simulink model "simulation_model_constcurrent"  (R2024b)
settings: Solver=VariableStepAuto  StartTime=0.0  StopTime=100  MaxStep=1/60  RelTol=1e-3  EnableMultiTasking=on
values from neighbouring files (symbols this model uses):
  c_f = c_f*Cb    [fun00_GFL_pu_2_normial.m]    (also in fun00_GFM_pu_2_normial.m)
  fb = 60    [case_data.m]    (also in sim_m_case1.m; sim_m_case1_bench.m; sim_m_case2.m; sim_m_case2_bench.m)
  ki_i = ki_i_pu*Vb_p_ph/Ib_p_ph    [fun00_GFL_pu_2_normial.m]    (also in fun00_GFM_pu_2_normial.m)
  ki_p = ki_p_pu/Sb*Ib_p_ph    [fun00_GFL_pu_2_normial.m]
  ki_pll = ki_pll/Vb_p_ph    [fun00_GFL_pu_2_normial.m]
  ki_q = ki_q_pu/Sb*Ib_p_ph    [fun00_GFL_pu_2_normial.m]
  kp_i = kp_i_pu*Vb_p_ph/Ib_p_ph    [fun00_GFL_pu_2_normial.m]    (also in fun00_GFM_pu_2_normial.m)
  kp_p = kp_p_pu/Sb*Ib_p_ph    [fun00_GFL_pu_2_normial.m]
  kp_pll = kp_pll/Vb_p_ph    [fun00_GFL_pu_2_normial.m]
  kp_q = kp_q_pu/Sb*Ib_p_ph    [fun00_GFL_pu_2_normial.m]
  l_f = l_f*Lb    [fun00_GFL_pu_2_normial.m]    (also in fun00_GFM_pu_2_normial.m)
  line = mpc.line    [sim_m_case1.m]    (also in sim_m_case1_bench.m; sim_m_case2.m = mpc.line*1.1; sim_m_case2_bench.m = mpc.line*1.1; sim_m_case2_sparse.m = mpc.line*1.1)
  pset = p_set_pu*Sb    [fun00_GFL_pu_2_normial.m]
  qset = q_set_pu*Sb    [fun00_GFL_pu_2_normial.m]
  r_f = r_f*Zb    [fun00_GFL_pu_2_normial.m]    (also in fun00_GFM_pu_2_normial.m)
  Sb = 100*10^6    (= 100000000)    [sim_m_case1.m]    (also in sim_m_case1_bench.m; sim_m_case2.m; sim_m_case2_bench.m; sim_m_case2_sparse.m)
  t_gfl = 35    [sim_m_case1.m]    (also in sim_m_case1_bench.m = 30; sim_m_case2.m; sim_m_case2_bench.m = 30; sim_m_case2_sparse.m)
  t_gfm = 30    [sim_m_case1.m]    (also in sim_m_case1_bench.m; sim_m_case2.m; sim_m_case2_bench.m; sim_m_case2_sparse.m)
  trans_l = mpc.trans_l    [sim_m_case1.m]    (also in sim_m_case1_bench.m; sim_m_case2.m; sim_m_case2_bench.m; sim_m_case2_sparse.m)
  Vb_gfm = 20*10^3    (= 20000)    [sim_m_case1.m]    (also in sim_m_case1_bench.m; sim_m_case2.m; sim_m_case2_bench.m; sim_m_case2_sparse.m)
  Vb_h = 230*10^3    (= 230000)    [sim_m_case1.m]    (also in sim_m_case1_bench.m; sim_m_case2.m; sim_m_case2_bench.m; sim_m_case2_sparse.m)
  Vdc = 3*Vb_p_ph    [fun00_GFL_pu_2_normial.m]    (also in fun00_GFM_pu_2_normial.m)
  wb = 2*pi*fb    (= 376.991118431)    [case_data.m]    (also in sim_m_case1.m; sim_m_case1_bench.m; sim_m_case2.m; sim_m_case2_bench.m)
undefined symbols (not defined in the file or in its folder): c_f_gfm, d_gfl, D_p_gfm, D_p_gfm_s, D_q_gfm, DiscIntNeverNeededParam, Init, Init_GFL, J_gfm, ki_i_gfm, ki_pll_s, ki_vc_gfm, kp_i_gfm, kp_pll_s, kp_vc_gfm, l_f_gfm, P_set_gfm, Q_set_gfm, r_f_gfm, Vb, Vdc_gfm, VSM
libraries: spsThreePhaseVIMeasurementLib x52, spsabctodq0Lib x48, slpidlib x42, spsThreePhaseSeriesRLCBranchLib x36, spsFirstOrderFilterLib x16, spsThreePhaseTransformerTwoWindingsLib x9, spsGroundLib x9, spsPowerPositiveSequenceLib x9, spsdq0toabcLib x9, spsUniversalBridgeLib x9, spsDCVoltageSourceLib x9, spsThreePhaseSourceLib x5
(part 7 of 8)

== system simulation_model_constcurrent/Area 3/INVERTER 7/GFM7/Current Lopp ==
  Vodq : Inport
  Icdq : Inport  Port=2
  i_ref_dq : Inport  Port=3
  theta : Inport  Port=4
  Demux : Demux  Outputs=2
  Demux1 : Demux  Outputs=2
  Demux4 : Demux  Outputs=2
  Gain : Gain  Gain=2/Vdcnorm
  Mux1 : Mux  Inputs=3
  Mux3 : Mux  Inputs=2
  Mux4 : Mux  Inputs=2
  PID Controller2 : slpidlib/PID Controller  Controller=PI  Form=Parallel  TimeDomain=Continuous-time  UseExternalTs=off  SampleTime=-1  IntegratorMethod=Forward Euler  FilterMethod=Forward Euler  ControllerParametersSource=internal  P=Current_P  I=Current_I  UseKiTs=off  D=0  UseExternalDerivativeSource=off  N=100  UseFilter=on  TunerSelectOption=Transfer Function Based (PID Tuner App)  InitialConditionSource=internal  InitialConditionForIntegrator=InitialV.Vcd-InitialV.Vod  InitialConditionForFilter=0  DifferentiatorICPrevScaledInput=0  ExternalReset=none  TrackingMode=off  Kt=1  LimitOutput=off  SatLimitsSource=internal  UpperSaturationLimit=inf  LowerSaturationLimit=-inf  LinearizeAsGain=on  AntiWindupMode=none  Kb=1  LimitIntegrator=off  UpperIntegratorSaturationLimit=inf  LowerIntegratorSaturationLimit=-inf  POutMin=[]  POutMax=[]  IOutMin=[]  IOutMax=[]  DOutMin=[]  DOutMax=[]  NOutMin=[]  NOutMax=[]  SumOutMin=[]  SumOutMax=[]  SaturationOutMin=[]  SaturationOutMax=[]  PParamMin=[]  PParamMax=[]  IParamMin=[]  IParamMax=[]  DParamMin=[]  DParamMax=[]  NParamMin=[]  NParamMax=[]  KbParamMin=[]  KbParamMax=[]  KtParamMin=[]  KtParamMax=[]  KbOutMin=[]  KbOutMax=[]  KtOutMin=[]  KtOutMax=[]  IntegratorOutMin=[]  IntegratorOutMax=[]  FilterOutMin=[]  FilterOutMax=[]  SumI1OutMin=[]  SumI1OutMax=[]  SumI2OutMin=[]  SumI2OutMax=[]  SumI3OutMin=[]  SumI3OutMax=[]  SumI4OutMin=[]  SumI4OutMax=[]  SumDOutMin=[]  SumDOutMax=[]  DifferentiatorOutMin=[]  DifferentiatorOutMax=[]  FilterDiffOutCoefMin=[]  FilterDiffOutCoefMax=[]  ReciprocalOutMin=[]  ReciprocalOutMax=[]  SumDenOutMin=[]  SumDenOutMax=[]  SumNumOutMin=[]  SumNumOutMax=[]  DivideOutMin=[]  DivideOutMax=[]  UdiffTsProdOutMin=[]  UdiffTsProdOutMax=[]  NTsProdOutMin=[]  NTsProdOutMax=[]  UintegralTsProdOutMin=[]  UintegralTsProdOutMax=[]  UngainTsProdOutMin=[]  UngainTsProdOutMax=[]  ClampingZeroOutDataTypeStr=Inherit: Inherit via back propagation  ClampingZeroOutMin=[]  ClampingZeroOutMax=[]  FilterDenConstantOutDataTypeStr=Inherit: Inherit via back propagation  FilterDenConstantOutMin=[]  FilterDenConstantOutMax=[]  PCopyOutDataTypeStr=Inherit: Inherit via back propagation  PCopyOutMin=[]  PCopyOutMax=[]  NCopyOutDataTypeStr=Inherit: Inherit via back propagation  NCopyOutMin=[]  NCopyOutMax=[]  IntegratorContinuousStateAttributes=''  IntegratorStateMustResolveToSignalObject=off  IntegratorRTWStateStorageClass=Auto  FilterContinuousStateAttributes=''  FilterStateMustResolveToSignalObject=off  FilterRTWStateStorageClass=Auto  ParallelPVariant=InternalParameters  IdealPVariant=Disabled  IVariant=InternalParameters  DVariant=Disabled  IntegratorVariant=Continuous  SatVariant=Disabled  AWVariant=Passthrough  PCopyVariant=Disabled  TRVariant=Disabled  FdbkBlocksVariant=Forward  IdealPFdbkVariant=Disabled  SatFdbkVariant=Disabled  DerivativeFilterVariant=Disabled  NVariant=Disabled  NCopyVariant=Disabled_SignalSpec  FilterICVariant=Disabled  IntegratorICVariant=InternalICs  ExternalResetVariant=Disabled  TRSumVariant=Passthrough  SumFdbkVariant=Disabled  SumVariant=Sum_PI  TsampFilterVariant=InternalTs  TsampNgainVariant=Passthrough  TsampIntegralVariant=Disabled_SignalSpec  ExternalSaturationOutDataTypeStr=Inherit: Same as second input  DerivativeSourceVariant=Disabled  PreIntVariant=InternalPreInt
  PID Controller3 : slpidlib/PID Controller  Controller=PI  Form=Parallel  TimeDomain=Continuous-time  UseExternalTs=off  SampleTime=-1  IntegratorMethod=Forward Euler  FilterMethod=Forward Euler  ControllerParametersSource=internal  P=Current_P  I=Current_I  UseKiTs=off  D=0  UseExternalDerivativeSource=off  N=100  UseFilter=on  TunerSelectOption=Transfer Function Based (PID Tuner App)  InitialConditionSource=internal  InitialConditionForIntegrator=InitialV.Vcq-InitialV.Voq  InitialConditionForFilter=0  DifferentiatorICPrevScaledInput=0  ExternalReset=none  TrackingMode=off  Kt=1  LimitOutput=off  SatLimitsSource=internal  UpperSaturationLimit=inf  LowerSaturationLimit=-inf  LinearizeAsGain=on  AntiWindupMode=none  Kb=1  LimitIntegrator=off  UpperIntegratorSaturationLimit=inf  LowerIntegratorSaturationLimit=-inf  POutMin=[]  POutMax=[]  IOutMin=[]  IOutMax=[]  DOutMin=[]  DOutMax=[]  NOutMin=[]  NOutMax=[]  SumOutMin=[]  SumOutMax=[]  SaturationOutMin=[]  SaturationOutMax=[]  PParamMin=[]  PParamMax=[]  IParamMin=[]  IParamMax=[]  DParamMin=[]  DParamMax=[]  NParamMin=[]  NParamMax=[]  KbParamMin=[]  KbParamMax=[]  KtParamMin=[]  KtParamMax=[]  KbOutMin=[]  KbOutMax=[]  KtOutMin=[]  KtOutMax=[]  IntegratorOutMin=[]  IntegratorOutMax=[]  FilterOutMin=[]  FilterOutMax=[]  SumI1OutMin=[]  SumI1OutMax=[]  SumI2OutMin=[]  SumI2OutMax=[]  SumI3OutMin=[]  SumI3OutMax=[]  SumI4OutMin=[]  SumI4OutMax=[]  SumDOutMin=[]  SumDOutMax=[]  DifferentiatorOutMin=[]  DifferentiatorOutMax=[]  FilterDiffOutCoefMin=[]  FilterDiffOutCoefMax=[]  ReciprocalOutMin=[]  ReciprocalOutMax=[]  SumDenOutMin=[]  SumDenOutMax=[]  SumNumOutMin=[]  SumNumOutMax=[]  DivideOutMin=[]  DivideOutMax=[]  UdiffTsProdOutMin=[]  UdiffTsProdOutMax=[]  NTsProdOutMin=[]  NTsProdOutMax=[]  UintegralTsProdOutMin=[]  UintegralTsProdOutMax=[]  UngainTsProdOutMin=[]  UngainTsProdOutMax=[]  ClampingZeroOutDataTypeStr=Inherit: Inherit via back propagation  ClampingZeroOutMin=[]  ClampingZeroOutMax=[]  FilterDenConstantOutDataTypeStr=Inherit: Inherit via back propagation  FilterDenConstantOutMin=[]  FilterDenConstantOutMax=[]  PCopyOutDataTypeStr=Inherit: Inherit via back propagation  PCopyOutMin=[]  PCopyOutMax=[]  NCopyOutDataTypeStr=Inherit: Inherit via back propagation  NCopyOutMin=[]  NCopyOutMax=[]  IntegratorContinuousStateAttributes=''  IntegratorStateMustResolveToSignalObject=off  IntegratorRTWStateStorageClass=Auto  FilterContinuousStateAttributes=''  FilterStateMustResolveToSignalObject=off  FilterRTWStateStorageClass=Auto  ParallelPVariant=InternalParameters  IdealPVariant=Disabled  IVariant=InternalParameters  DVariant=Disabled  IntegratorVariant=Continuous  SatVariant=Disabled  AWVariant=Passthrough  PCopyVariant=Disabled  TRVariant=Disabled  FdbkBlocksVariant=Forward  IdealPFdbkVariant=Disabled  SatFdbkVariant=Disabled  DerivativeFilterVariant=Disabled  NVariant=Disabled  NCopyVariant=Disabled_SignalSpec  FilterICVariant=Disabled  IntegratorICVariant=InternalICs  ExternalResetVariant=Disabled  TRSumVariant=Passthrough  SumFdbkVariant=Disabled  SumVariant=Sum_PI  TsampFilterVariant=InternalTs  TsampNgainVariant=Passthrough  TsampIntegralVariant=Disabled_SignalSpec  ExternalSaturationOutDataTypeStr=Inherit: Same as second input  DerivativeSourceVariant=Disabled  PreIntVariant=InternalPreInt
  Scope : Scope  NumInputPorts=2
  Sum2 : Sum  Inputs=-+|
  Sum3 : Sum  Inputs=|+-
  Sum6 : Sum  Inputs=++|
  Sum7 : Sum  Inputs=|++
  Unit Delay1 : UnitDelay  SampleTime=-1  HasFrameUpgradeWarning=on
  V0 : Constant  Value=0
  VSG_ref : Scope  NumInputPorts=2
  dq0 to abc : spsdq0toabcLib/dq0 to abc  Alignment=Aligned with phase A axis
  电流对比 : Scope  NumInputPorts=2
  VSG_Uref : Outport
  wires:
  Mux4/1 -> 电流对比/1
  Mux1/1 -> Scope/1, Gain/1
  Vodq/1 -> Demux1/1
  Demux1/1 -> [Vod]
  Demux1/2 -> [Voq]
  Demux4/1 -> [Icd]
  Icdq/1 -> Demux4/1
  Demux4/2 -> [Icq]
  [Icd] -> Mux4/2
  [Icdref] -> Mux4/1
  [Icqref] -> Mux3/1
  [Icq] -> Mux3/2
  Mux3/1 -> 电流对比/2
  [Icd] -> Sum2/1
  Sum2/1 -> PID Controller2/1
  Sum3/1 -> PID Controller3/1
  V0/1 -> Mux1/3
  theta/1 -> dq0 to abc/2
  PID Controller2/1 -> Sum6/2
  PID Controller3/1 -> Sum7/1
  Sum7/1 -> Mux1/2, VSG_ref/2
  Sum6/1 -> Mux1/1, VSG_ref/1
  dq0 to abc/1 -> Unit Delay1/1
  [Icq] -> Sum3/2
  [Icdref] -> Sum2/2
  [Icqref] -> Sum3/1
  Unit Delay1/1 -> VSG_Uref/1
  Gain/1 -> dq0 to abc/1, Scope/2
  i_ref_dq/1 -> Demux/1
  Demux/1 -> [Icdref]
  Demux/2 -> [Icqref]
  [Vod] -> Sum6/1
  [Voq] -> Sum7/2

== system simulation_model_constcurrent/Area 3/INVERTER 7/GFM7/Measurement ==
  Vabc_s0 : Inport
  Iabc_s0 : Inport  Port=2
  Iabc_s2 : Inport  Port=3
  theta : Inport  Port=4
  " " : spsPowerPositiveSequenceLib/Power (Positive-Sequence)  Freq=fbnorm  Vinit=[0, 0]  Iinit=[0, 0]  Ts=0
  Add1 : Sum  Inputs=-+
  Add2 : Sum
  Demux : Demux  Outputs=2
  Demux1 : Demux  Outputs=2
  Fcn : Fcn  Expr=sqrt(u(1)^2 + u(2)^2)
  Gain : Gain
  Gain{1,3..5} (4 alike) : Gain  Gain=3/2
  Gain2 : Gain
  Mux : Mux  Inputs=2
  Mux1 : Mux  Inputs=2
  Mux2 : Mux  Inputs=2
  Product{,1..3} (4 alike) : Product
  Scope{,1..3} (4 alike) : Scope
  Selector : Selector  InputPortWidth=3  IndexOptions=Index vector (dialog)  Indices=[1 2]  OutputSizes=2
  Selector1 : Selector  InputPortWidth=3  IndexOptions=Index vector (dialog)  Indices=[1 2]  OutputSizes=2
  Selector2 : Selector  InputPortWidth=3  IndexOptions=Index vector (dialog)  Indices=[1 2]  OutputSizes=2
  True : Scope
  True P : Scope
  True Q : Scope
  abc to dq0 : spsabctodq0Lib/abc to dq0  Alignment=Aligned with phase A axis
  abc to dq3 : spsabctodq0Lib/abc to dq0  Alignment=Aligned with phase A axis
  abc to dq4 : spsabctodq0Lib/abc to dq0  Alignment=Aligned with phase A axis
  P : Outport
  Q : Outport  Port=2
  Vodq : Outport  Port=3
  Icdq : Outport  Port=4
  Vrms : Outport  Port=5
  wires:
  abc to dq0/1 -> Fcn/1, Selector/1
  theta/1 -> abc to dq4/2, abc to dq3/2, abc to dq0/2
  Add2/1 -> Mux1/2, P/1, Scope2/1
  [Voq] -> Product3/1
  Iabc_s0/1 -> " "/2, abc to dq3/1
  Iabc_s2/1 -> abc to dq4/1
  [Iod] -> Product/2
  [Vod] -> Product1/1
  Selector/1 -> Vodq/1, Demux/1, Scope/1
  [Voq] -> Product2/1
  abc to dq4/1 -> Selector2/1
  [Vod] -> Product/1
  Demux/1 -> [Vod]
  Vabc_s0/1 -> " "/1, abc to dq0/1
  Mux2/1 -> True Q/1
  Fcn/1 -> Vrms/1
  Add1/1 -> Mux2/2, Q/1, Scope3/1
  Mux1/1 -> True P/1
  Selector1/1 -> Demux1/1, Scope1/1
  abc to dq3/1 -> Selector1/1
  Product3/1 -> Gain5/1
  [Ioq] -> Product1/2
  [Iod] -> Product3/2
  Product1/1 -> Gain4/1
  Demux1/2 -> [Ioq]
  Demux1/1 -> [Iod]
  Demux/2 -> [Voq]
  Mux/1 -> True/1
  [Ioq] -> Product2/2
  Selector2/1 -> Icdq/1
  Product2/1 -> Gain3/1
  Product/1 -> Gain1/1
  " "/2 -> Gain2/1
  " "/1 -> Gain/1
  Gain/1 -> Mux1/1, Mux/1
  Gain2/1 -> Mux2/1, Mux/2
  Gain1/1 -> Add2/1
  Gain3/1 -> Add2/2
  Gain4/1 -> Add1/1
  Gain5/1 -> Add1/2

== system simulation_model_constcurrent/Area 3/INVERTER 7/GFM7/Subsystem3 ==
  theta : Inport
  Vabc : Inport  Port=2
  Iabc : Inport  Port=3
  abc to dq1 : spsabctodq0Lib/abc to dq0  Alignment=Aligned with phase A axis
  abc to dq2 : spsabctodq0Lib/abc to dq0  Alignment=Aligned with phase A axis
  Vdq0 : Outport
  Idq0 : Outport  Port=2
  wires:
  Iabc/1 -> abc to dq2/1
  theta/1 -> abc to dq2/2, abc to dq1/2
  abc to dq1/1 -> Vdq0/1
  Vabc/1 -> abc to dq1/1
  abc to dq2/1 -> Idq0/1

== system simulation_model_constcurrent/Area 3/INVERTER 7/GFM7/VSM control ==
  P : Inport
  P_set : Inport  Port=2
  Q : Inport  Port=3
  Q_set : Inport  Port=4
  Clock : Clock
  Clock1 : Clock
  Constant : Constant  Value=2*pi*fbnorm
  Constant1 : Constant  Value=0
  Constant2 : Constant  Value=Vbnorm/sqrt(3)*sqrt(2)
  Constant3 : Constant  Value=2*pi
  Constant5 : Constant  Value=2*pi*fbnorm
  Constant6 : Constant  Value=VSM(7)
  First-Order Filter : spsFirstOrderFilterLib/First-Order Filter  FilterType=Lowpass  Tc=0.08  Ts=0  Initialize=on  Vac_Init=[0, 0, 0]  Vdc_Init=wb  PlotResponse=off  FreqRange="[0,  200,  1]"
  First-Order Filter1 : spsFirstOrderFilterLib/First-Order Filter  FilterType=Lowpass  Tc=0.01  Ts=0  Initialize=on  Vac_Init=[0, 0, 0]  Vdc_Init=Vbnorm/sqrt(3)*sqrt(2)  PlotResponse=off  FreqRange="[0,  200,  1]"
  Gain : Gain  Gain=1/Dq
  Gain1 : Gain  Gain=Dp
  Gain2 : Gain  Gain=D_p_gfm_s(7)
  Gain4 : Gain  Gain=1/Dp
  Gain5 : Gain  Gain=1/D_p_gfm_s(7)
  Gain6 : Gain  Gain=1/J
  Integrator : Integrator  InitialCondition=2*pi*fbnorm
  Integrator1 : Integrator
  Integrator2 : Integrator  InitialCondition=InitialV.theta0
  Mod : Math  Operator=mod
  Multiport Switch : MultiPortSwitch  Inputs=2  SaturateOnIntegerOverflow=off  InputSameDT=off
  Mux : Mux  Inputs=2
  Sum : Sum  Inputs=-|+|-
  Sum1 : Sum  Inputs=-|+
  Sum2 : Sum  Inputs=-+
  Sum3 : Sum  Inputs=+-|
  Sum4 : Sum  Inputs=-|+
  Sum5 : Sum  Inputs=+-|
  Switch : Switch  Threshold=t_gfm  SaturateOnIntegerOverflow=off  InputSameDT=off
  Switch1 : Switch  Threshold=t_gfm  SaturateOnIntegerOverflow=off  InputSameDT=off
  w_ref : Outport  VectorParamsAs1DForOutWhenUnconnected=off
  theta_ref : Outport  Port=2  VectorParamsAs1DForOutWhenUnconnected=off
  Vodq_ref : Outport  Port=3  VectorParamsAs1DForOutWhenUnconnected=off
  theta_output : Outport  Port=4
  theta0 : Outport  Port=5
  wires:
  Constant/1 -> Sum2/1
  Sum/1 -> Gain6/1
  Switch/1 -> [d_output]
  [d_output] -> Sum/1
  Constant2/1 -> Sum3/1
  Mod/1 -> theta_ref/1
  Multiport Switch/1 -> [switch_w]
  Q_set/1 -> Sum1/1
  Mux/1 -> Vodq_ref/1
  Q/1 -> Sum1/2
  Sum1/1 -> Gain/1
  Gain2/1 -> Switch/1
  Integrator2/1 -> theta_output/1, Mod/1  "theta"
  Integrator/1 -> Sum2/2, [vsm_output]  "w"
  Sum2/1 -> [d_input], Integrator1/1
  Constant3/1 -> Mod/2
  Clock/1 -> Switch/2
  [d_output1] -> Sum5/2
  [d_input] -> Gain2/1
  [d_input] -> Gain1/1
  [droop_output] -> Multiport Switch/3
  Sum3/1 -> First-Order Filter1/1
  Constant5/1 -> Sum5/1
  Sum4/1 -> [d_input1]
  Gain6/1 -> Integrator/1
  P_set/1 -> Sum4/1, Sum/2
  Integrator1/1 -> theta0/1
  Constant1/1 -> Mux/2
  Sum5/1 -> First-Order Filter/1
  [vsm_output] -> Multiport Switch/2
  Gain1/1 -> Switch/3
  [switch_w] -> Integrator2/1, w_ref/1
  P/1 -> Sum4/2, Sum/3
  Constant6/1 -> Multiport Switch/1
  First-Order Filter/1 -> [droop_output]
  Gain4/1 -> Switch1/3
  Clock1/1 -> Switch1/2
  [d_input1] -> Gain4/1
  Gain5/1 -> Switch1/1
  [d_input1] -> Gain5/1
  Switch1/1 -> [d_output1]
  Gain/1 -> Sum3/2
  First-Order Filter1/1 -> Mux/1

== system simulation_model_constcurrent/Area 3/INVERTER 7/GFM7/Voltage Loop ==
  v_ref_dq : Inport
  vo_dq : Inport  Port=2
  Demux : Demux  Outputs=2
  Demux1 : Demux  Outputs=2
  Mux : Mux  Inputs=2
  PID Controller : slpidlib/PID Controller  Controller=PI  Form=Parallel  TimeDomain=Continuous-time  UseExternalTs=off  SampleTime=-1  IntegratorMethod=Forward Euler  FilterMethod=Forward Euler  ControllerParametersSource=internal  P=Voltage_P  I=Voltage_I  UseKiTs=off  D=0  UseExternalDerivativeSource=off  N=100  UseFilter=on  TunerSelectOption=Transfer Function Based (PID Tuner App)  InitialConditionSource=internal  InitialConditionForIntegrator=InitialV.Icd  InitialConditionForFilter=0  DifferentiatorICPrevScaledInput=0  ExternalReset=none  TrackingMode=off  Kt=1  LimitOutput=off  SatLimitsSource=internal  UpperSaturationLimit=inf  LowerSaturationLimit=-inf  LinearizeAsGain=on  AntiWindupMode=none  Kb=1  LimitIntegrator=off  UpperIntegratorSaturationLimit=inf  LowerIntegratorSaturationLimit=-inf  POutMin=[]  POutMax=[]  IOutMin=[]  IOutMax=[]  DOutMin=[]  DOutMax=[]  NOutMin=[]  NOutMax=[]  SumOutMin=[]  SumOutMax=[]  SaturationOutMin=[]  SaturationOutMax=[]  PParamMin=[]  PParamMax=[]  IParamMin=[]  IParamMax=[]  DParamMin=[]  DParamMax=[]  NParamMin=[]  NParamMax=[]  KbParamMin=[]  KbParamMax=[]  KtParamMin=[]  KtParamMax=[]  KbOutMin=[]  KbOutMax=[]  KtOutMin=[]  KtOutMax=[]  IntegratorOutMin=[]  IntegratorOutMax=[]  FilterOutMin=[]  FilterOutMax=[]  SumI1OutMin=[]  SumI1OutMax=[]  SumI2OutMin=[]  SumI2OutMax=[]  SumI3OutMin=[]  SumI3OutMax=[]  SumI4OutMin=[]  SumI4OutMax=[]  SumDOutMin=[]  SumDOutMax=[]  DifferentiatorOutMin=[]  DifferentiatorOutMax=[]  FilterDiffOutCoefMin=[]  FilterDiffOutCoefMax=[]  ReciprocalOutMin=[]  ReciprocalOutMax=[]  SumDenOutMin=[]  SumDenOutMax=[]  SumNumOutMin=[]  SumNumOutMax=[]  DivideOutMin=[]  DivideOutMax=[]  UdiffTsProdOutMin=[]  UdiffTsProdOutMax=[]  NTsProdOutMin=[]  NTsProdOutMax=[]  UintegralTsProdOutMin=[]  UintegralTsProdOutMax=[]  UngainTsProdOutMin=[]  UngainTsProdOutMax=[]  ClampingZeroOutDataTypeStr=Inherit: Inherit via back propagation  ClampingZeroOutMin=[]  ClampingZeroOutMax=[]  FilterDenConstantOutDataTypeStr=Inherit: Inherit via back propagation  FilterDenConstantOutMin=[]  FilterDenConstantOutMax=[]  PCopyOutDataTypeStr=Inherit: Inherit via back propagation  PCopyOutMin=[]  PCopyOutMax=[]  NCopyOutDataTypeStr=Inherit: Inherit via back propagation  NCopyOutMin=[]  NCopyOutMax=[]  IntegratorContinuousStateAttributes=''  IntegratorStateMustResolveToSignalObject=off  IntegratorRTWStateStorageClass=Auto  FilterContinuousStateAttributes=''  FilterStateMustResolveToSignalObject=off  FilterRTWStateStorageClass=Auto  ParallelPVariant=InternalParameters  IdealPVariant=Disabled  IVariant=InternalParameters  DVariant=Disabled  IntegratorVariant=Continuous  SatVariant=Disabled  AWVariant=Passthrough  PCopyVariant=Disabled  TRVariant=Disabled  FdbkBlocksVariant=Forward  IdealPFdbkVariant=Disabled  SatFdbkVariant=Disabled  DerivativeFilterVariant=Disabled  NVariant=Disabled  NCopyVariant=Disabled_SignalSpec  FilterICVariant=Disabled  IntegratorICVariant=InternalICs  ExternalResetVariant=Disabled  TRSumVariant=Passthrough  SumFdbkVariant=Disabled  SumVariant=Sum_PI  TsampFilterVariant=InternalTs  TsampNgainVariant=Passthrough  TsampIntegralVariant=Disabled_SignalSpec  ExternalSaturationOutDataTypeStr=Inherit: Same as second input  DerivativeSourceVariant=Disabled  PreIntVariant=InternalPreInt
  PID Controller1 : slpidlib/PID Controller  Controller=PI  Form=Parallel  TimeDomain=Continuous-time  UseExternalTs=off  SampleTime=-1  IntegratorMethod=Forward Euler  FilterMethod=Forward Euler  ControllerParametersSource=internal  P=Voltage_P  I=Voltage_I  UseKiTs=off  D=0  UseExternalDerivativeSource=off  N=100  UseFilter=on  TunerSelectOption=Transfer Function Based (PID Tuner App)  InitialConditionSource=internal  InitialConditionForIntegrator=InitialV.Icq  InitialConditionForFilter=0  DifferentiatorICPrevScaledInput=0  ExternalReset=none  TrackingMode=off  Kt=1  LimitOutput=off  SatLimitsSource=internal  UpperSaturationLimit=inf  LowerSaturationLimit=-inf  LinearizeAsGain=on  AntiWindupMode=none  Kb=1  LimitIntegrator=off  UpperIntegratorSaturationLimit=inf  LowerIntegratorSaturationLimit=-inf  POutMin=[]  POutMax=[]  IOutMin=[]  IOutMax=[]  DOutMin=[]  DOutMax=[]  NOutMin=[]  NOutMax=[]  SumOutMin=[]  SumOutMax=[]  SaturationOutMin=[]  SaturationOutMax=[]  PParamMin=[]  PParamMax=[]  IParamMin=[]  IParamMax=[]  DParamMin=[]  DParamMax=[]  NParamMin=[]  NParamMax=[]  KbParamMin=[]  KbParamMax=[]  KtParamMin=[]  KtParamMax=[]  KbOutMin=[]  KbOutMax=[]  KtOutMin=[]  KtOutMax=[]  IntegratorOutMin=[]  IntegratorOutMax=[]  FilterOutMin=[]  FilterOutMax=[]  SumI1OutMin=[]  SumI1OutMax=[]  SumI2OutMin=[]  SumI2OutMax=[]  SumI3OutMin=[]  SumI3OutMax=[]  SumI4OutMin=[]  SumI4OutMax=[]  SumDOutMin=[]  SumDOutMax=[]  DifferentiatorOutMin=[]  DifferentiatorOutMax=[]  FilterDiffOutCoefMin=[]  FilterDiffOutCoefMax=[]  ReciprocalOutMin=[]  ReciprocalOutMax=[]  SumDenOutMin=[]  SumDenOutMax=[]  SumNumOutMin=[]  SumNumOutMax=[]  DivideOutMin=[]  DivideOutMax=[]  UdiffTsProdOutMin=[]  UdiffTsProdOutMax=[]  NTsProdOutMin=[]  NTsProdOutMax=[]  UintegralTsProdOutMin=[]  UintegralTsProdOutMax=[]  UngainTsProdOutMin=[]  UngainTsProdOutMax=[]  ClampingZeroOutDataTypeStr=Inherit: Inherit via back propagation  ClampingZeroOutMin=[]  ClampingZeroOutMax=[]  FilterDenConstantOutDataTypeStr=Inherit: Inherit via back propagation  FilterDenConstantOutMin=[]  FilterDenConstantOutMax=[]  PCopyOutDataTypeStr=Inherit: Inherit via back propagation  PCopyOutMin=[]  PCopyOutMax=[]  NCopyOutDataTypeStr=Inherit: Inherit via back propagation  NCopyOutMin=[]  NCopyOutMax=[]  IntegratorContinuousStateAttributes=''  IntegratorStateMustResolveToSignalObject=off  IntegratorRTWStateStorageClass=Auto  FilterContinuousStateAttributes=''  FilterStateMustResolveToSignalObject=off  FilterRTWStateStorageClass=Auto  ParallelPVariant=InternalParameters  IdealPVariant=Disabled  IVariant=InternalParameters  DVariant=Disabled  IntegratorVariant=Continuous  SatVariant=Disabled  AWVariant=Passthrough  PCopyVariant=Disabled  TRVariant=Disabled  FdbkBlocksVariant=Forward  IdealPFdbkVariant=Disabled  SatFdbkVariant=Disabled  DerivativeFilterVariant=Disabled  NVariant=Disabled  NCopyVariant=Disabled_SignalSpec  FilterICVariant=Disabled  IntegratorICVariant=InternalICs  ExternalResetVariant=Disabled  TRSumVariant=Passthrough  SumFdbkVariant=Disabled  SumVariant=Sum_PI  TsampFilterVariant=InternalTs  TsampNgainVariant=Passthrough  TsampIntegralVariant=Disabled_SignalSpec  ExternalSaturationOutDataTypeStr=Inherit: Same as second input  DerivativeSourceVariant=Disabled  PreIntVariant=InternalPreInt
  Sum : Sum  Inputs=|+-
  Sum1 : Sum  Inputs=|+-
  i_ref_dq : Outport  VectorParamsAs1DForOutWhenUnconnected=off
  wires:
  Mux/1 -> i_ref_dq/1
  v_ref_dq/1 -> Demux/1
  vo_dq/1 -> Demux1/1
  Demux/1 -> [vo_ref_d]
  Demux/2 -> [vo_ref_q]
  Demux1/1 -> [vo_d]
  Demux1/2 -> [vo_q]
  Sum/1 -> PID Controller/1
  [vo_d] -> Sum/2
  Sum1/1 -> PID Controller1/1
  [vo_q] -> Sum1/2
  PID Controller/1 -> Mux/1
  PID Controller1/1 -> Mux/2
  [vo_ref_d] -> Sum/1
  [vo_ref_q] -> Sum1/1

== system simulation_model_constcurrent/Area 3/INVERTER 8/GFM8/Current Lopp ==
  Vodq : Inport
  Icdq : Inport  Port=2
  i_ref_dq : Inport  Port=3
  theta : Inport  Port=4
  Demux : Demux  Outputs=2
  Demux1 : Demux  Outputs=2
  Demux4 : Demux  Outputs=2
  Gain : Gain  Gain=2/Vdcnorm
  Mux1 : Mux  Inputs=3
  Mux3 : Mux  Inputs=2
  Mux4 : Mux  Inputs=2
  PID Controller2 : slpidlib/PID Controller  Controller=PI  Form=Parallel  TimeDomain=Continuous-time  UseExternalTs=off  SampleTime=-1  IntegratorMethod=Forward Euler  FilterMethod=Forward Euler  ControllerParametersSource=internal  P=Current_P  I=Current_I  UseKiTs=off  D=0  UseExternalDerivativeSource=off  N=100  UseFilter=on  TunerSelectOption=Transfer Function Based (PID Tuner App)  InitialConditionSource=internal  InitialConditionForIntegrator=InitialV.Vcd-InitialV.Vod  InitialConditionForFilter=0  DifferentiatorICPrevScaledInput=0  ExternalReset=none  TrackingMode=off  Kt=1  LimitOutput=off  SatLimitsSource=internal  UpperSaturationLimit=inf  LowerSaturationLimit=-inf  LinearizeAsGain=on  AntiWindupMode=none  Kb=1  LimitIntegrator=off  UpperIntegratorSaturationLimit=inf  LowerIntegratorSaturationLimit=-inf  POutMin=[]  POutMax=[]  IOutMin=[]  IOutMax=[]  DOutMin=[]  DOutMax=[]  NOutMin=[]  NOutMax=[]  SumOutMin=[]  SumOutMax=[]  SaturationOutMin=[]  SaturationOutMax=[]  PParamMin=[]  PParamMax=[]  IParamMin=[]  IParamMax=[]  DParamMin=[]  DParamMax=[]  NParamMin=[]  NParamMax=[]  KbParamMin=[]  KbParamMax=[]  KtParamMin=[]  KtParamMax=[]  KbOutMin=[]  KbOutMax=[]  KtOutMin=[]  KtOutMax=[]  IntegratorOutMin=[]  IntegratorOutMax=[]  FilterOutMin=[]  FilterOutMax=[]  SumI1OutMin=[]  SumI1OutMax=[]  SumI2OutMin=[]  SumI2OutMax=[]  SumI3OutMin=[]  SumI3OutMax=[]  SumI4OutMin=[]  SumI4OutMax=[]  SumDOutMin=[]  SumDOutMax=[]  DifferentiatorOutMin=[]  DifferentiatorOutMax=[]  FilterDiffOutCoefMin=[]  FilterDiffOutCoefMax=[]  ReciprocalOutMin=[]  ReciprocalOutMax=[]  SumDenOutMin=[]  SumDenOutMax=[]  SumNumOutMin=[]  SumNumOutMax=[]  DivideOutMin=[]  DivideOutMax=[]  UdiffTsProdOutMin=[]  UdiffTsProdOutMax=[]  NTsProdOutMin=[]  NTsProdOutMax=[]  UintegralTsProdOutMin=[]  UintegralTsProdOutMax=[]  UngainTsProdOutMin=[]  UngainTsProdOutMax=[]  ClampingZeroOutDataTypeStr=Inherit: Inherit via back propagation  ClampingZeroOutMin=[]  ClampingZeroOutMax=[]  FilterDenConstantOutDataTypeStr=Inherit: Inherit via back propagation  FilterDenConstantOutMin=[]  FilterDenConstantOutMax=[]  PCopyOutDataTypeStr=Inherit: Inherit via back propagation  PCopyOutMin=[]  PCopyOutMax=[]  NCopyOutDataTypeStr=Inherit: Inherit via back propagation  NCopyOutMin=[]  NCopyOutMax=[]  IntegratorContinuousStateAttributes=''  IntegratorStateMustResolveToSignalObject=off  IntegratorRTWStateStorageClass=Auto  FilterContinuousStateAttributes=''  FilterStateMustResolveToSignalObject=off  FilterRTWStateStorageClass=Auto  ParallelPVariant=InternalParameters  IdealPVariant=Disabled  IVariant=InternalParameters  DVariant=Disabled  IntegratorVariant=Continuous  SatVariant=Disabled  AWVariant=Passthrough  PCopyVariant=Disabled  TRVariant=Disabled  FdbkBlocksVariant=Forward  IdealPFdbkVariant=Disabled  SatFdbkVariant=Disabled  DerivativeFilterVariant=Disabled  NVariant=Disabled  NCopyVariant=Disabled_SignalSpec  FilterICVariant=Disabled  IntegratorICVariant=InternalICs  ExternalResetVariant=Disabled  TRSumVariant=Passthrough  SumFdbkVariant=Disabled  SumVariant=Sum_PI  TsampFilterVariant=InternalTs  TsampNgainVariant=Passthrough  TsampIntegralVariant=Disabled_SignalSpec  ExternalSaturationOutDataTypeStr=Inherit: Same as second input  DerivativeSourceVariant=Disabled  PreIntVariant=InternalPreInt
  PID Controller3 : slpidlib/PID Controller  Controller=PI  Form=Parallel  TimeDomain=Continuous-time  UseExternalTs=off  SampleTime=-1  IntegratorMethod=Forward Euler  FilterMethod=Forward Euler  ControllerParametersSource=internal  P=Current_P  I=Current_I  UseKiTs=off  D=0  UseExternalDerivativeSource=off  N=100  UseFilter=on  TunerSelectOption=Transfer Function Based (PID Tuner App)  InitialConditionSource=internal  InitialConditionForIntegrator=InitialV.Vcq-InitialV.Voq  InitialConditionForFilter=0  DifferentiatorICPrevScaledInput=0  ExternalReset=none  TrackingMode=off  Kt=1  LimitOutput=off  SatLimitsSource=internal  UpperSaturationLimit=inf  LowerSaturationLimit=-inf  LinearizeAsGain=on  AntiWindupMode=none  Kb=1  LimitIntegrator=off  UpperIntegratorSaturationLimit=inf  LowerIntegratorSaturationLimit=-inf  POutMin=[]  POutMax=[]  IOutMin=[]  IOutMax=[]  DOutMin=[]  DOutMax=[]  NOutMin=[]  NOutMax=[]  SumOutMin=[]  SumOutMax=[]  SaturationOutMin=[]  SaturationOutMax=[]  PParamMin=[]  PParamMax=[]  IParamMin=[]  IParamMax=[]  DParamMin=[]  DParamMax=[]  NParamMin=[]  NParamMax=[]  KbParamMin=[]  KbParamMax=[]  KtParamMin=[]  KtParamMax=[]  KbOutMin=[]  KbOutMax=[]  KtOutMin=[]  KtOutMax=[]  IntegratorOutMin=[]  IntegratorOutMax=[]  FilterOutMin=[]  FilterOutMax=[]  SumI1OutMin=[]  SumI1OutMax=[]  SumI2OutMin=[]  SumI2OutMax=[]  SumI3OutMin=[]  SumI3OutMax=[]  SumI4OutMin=[]  SumI4OutMax=[]  SumDOutMin=[]  SumDOutMax=[]  DifferentiatorOutMin=[]  DifferentiatorOutMax=[]  FilterDiffOutCoefMin=[]  FilterDiffOutCoefMax=[]  ReciprocalOutMin=[]  ReciprocalOutMax=[]  SumDenOutMin=[]  SumDenOutMax=[]  SumNumOutMin=[]  SumNumOutMax=[]  DivideOutMin=[]  DivideOutMax=[]  UdiffTsProdOutMin=[]  UdiffTsProdOutMax=[]  NTsProdOutMin=[]  NTsProdOutMax=[]  UintegralTsProdOutMin=[]  UintegralTsProdOutMax=[]  UngainTsProdOutMin=[]  UngainTsProdOutMax=[]  ClampingZeroOutDataTypeStr=Inherit: Inherit via back propagation  ClampingZeroOutMin=[]  ClampingZeroOutMax=[]  FilterDenConstantOutDataTypeStr=Inherit: Inherit via back propagation  FilterDenConstantOutMin=[]  FilterDenConstantOutMax=[]  PCopyOutDataTypeStr=Inherit: Inherit via back propagation  PCopyOutMin=[]  PCopyOutMax=[]  NCopyOutDataTypeStr=Inherit: Inherit via back propagation  NCopyOutMin=[]  NCopyOutMax=[]  IntegratorContinuousStateAttributes=''  IntegratorStateMustResolveToSignalObject=off  IntegratorRTWStateStorageClass=Auto  FilterContinuousStateAttributes=''  FilterStateMustResolveToSignalObject=off  FilterRTWStateStorageClass=Auto  ParallelPVariant=InternalParameters  IdealPVariant=Disabled  IVariant=InternalParameters  DVariant=Disabled  IntegratorVariant=Continuous  SatVariant=Disabled  AWVariant=Passthrough  PCopyVariant=Disabled  TRVariant=Disabled  FdbkBlocksVariant=Forward  IdealPFdbkVariant=Disabled  SatFdbkVariant=Disabled  DerivativeFilterVariant=Disabled  NVariant=Disabled  NCopyVariant=Disabled_SignalSpec  FilterICVariant=Disabled  IntegratorICVariant=InternalICs  ExternalResetVariant=Disabled  TRSumVariant=Passthrough  SumFdbkVariant=Disabled  SumVariant=Sum_PI  TsampFilterVariant=InternalTs  TsampNgainVariant=Passthrough  TsampIntegralVariant=Disabled_SignalSpec  ExternalSaturationOutDataTypeStr=Inherit: Same as second input  DerivativeSourceVariant=Disabled  PreIntVariant=InternalPreInt
  Scope : Scope  NumInputPorts=2
  Sum2 : Sum  Inputs=-+|
  Sum3 : Sum  Inputs=|+-
  Sum6 : Sum  Inputs=++|
  Sum7 : Sum  Inputs=|++
  Unit Delay1 : UnitDelay  SampleTime=-1  HasFrameUpgradeWarning=on
  V0 : Constant  Value=0
  VSG_ref : Scope  NumInputPorts=2
  dq0 to abc : spsdq0toabcLib/dq0 to abc  Alignment=Aligned with phase A axis
  电流对比 : Scope  NumInputPorts=2
  VSG_Uref : Outport
  wires:
  Mux4/1 -> 电流对比/1
  Mux1/1 -> Scope/1, Gain/1
  Vodq/1 -> Demux1/1
  Demux1/1 -> [Vod]
  Demux1/2 -> [Voq]
  Demux4/1 -> [Icd]
  Icdq/1 -> Demux4/1
  Demux4/2 -> [Icq]
  [Icd] -> Mux4/2
  [Icdref] -> Mux4/1
  [Icqref] -> Mux3/1
  [Icq] -> Mux3/2
  Mux3/1 -> 电流对比/2
  [Icd] -> Sum2/1
  Sum2/1 -> PID Controller2/1
  Sum3/1 -> PID Controller3/1
  V0/1 -> Mux1/3
  theta/1 -> dq0 to abc/2
  PID Controller2/1 -> Sum6/2
  PID Controller3/1 -> Sum7/1
  Sum7/1 -> Mux1/2, VSG_ref/2
  Sum6/1 -> Mux1/1, VSG_ref/1
  dq0 to abc/1 -> Unit Delay1/1
  [Icq] -> Sum3/2
  [Icdref] -> Sum2/2
  [Icqref] -> Sum3/1
  Unit Delay1/1 -> VSG_Uref/1
  Gain/1 -> dq0 to abc/1, Scope/2
  i_ref_dq/1 -> Demux/1
  Demux/1 -> [Icdref]
  Demux/2 -> [Icqref]
  [Vod] -> Sum6/1
  [Voq] -> Sum7/2

== system simulation_model_constcurrent/Area 3/INVERTER 8/GFM8/Measurement ==
  Vabc_s0 : Inport
  Iabc_s0 : Inport  Port=2
  Iabc_s2 : Inport  Port=3
  theta : Inport  Port=4
  " " : spsPowerPositiveSequenceLib/Power (Positive-Sequence)  Freq=fbnorm  Vinit=[0, 0]  Iinit=[0, 0]  Ts=0
  Add1 : Sum  Inputs=-+
  Add2 : Sum
  Demux : Demux  Outputs=2
  Demux1 : Demux  Outputs=2
  Fcn : Fcn  Expr=sqrt(u(1)^2 + u(2)^2)
  Gain : Gain
  Gain{1,3..5} (4 alike) : Gain  Gain=3/2
  Gain2 : Gain
  Mux : Mux  Inputs=2
  Mux1 : Mux  Inputs=2
  Mux2 : Mux  Inputs=2
  Product{,1..3} (4 alike) : Product
  Scope{,1..3} (4 alike) : Scope
  Selector : Selector  InputPortWidth=3  IndexOptions=Index vector (dialog)  Indices=[1 2]  OutputSizes=2
  Selector1 : Selector  InputPortWidth=3  IndexOptions=Index vector (dialog)  Indices=[1 2]  OutputSizes=2
  Selector2 : Selector  InputPortWidth=3  IndexOptions=Index vector (dialog)  Indices=[1 2]  OutputSizes=2
  True : Scope
  True P : Scope
  True Q : Scope
  abc to dq0 : spsabctodq0Lib/abc to dq0  Alignment=Aligned with phase A axis
  abc to dq3 : spsabctodq0Lib/abc to dq0  Alignment=Aligned with phase A axis
  abc to dq4 : spsabctodq0Lib/abc to dq0  Alignment=Aligned with phase A axis
  P : Outport
  Q : Outport  Port=2
  Vodq : Outport  Port=3
  Icdq : Outport  Port=4
  Vrms : Outport  Port=5
  wires:
  abc to dq0/1 -> Fcn/1, Selector/1
  theta/1 -> abc to dq4/2, abc to dq3/2, abc to dq0/2
  Add2/1 -> Mux1/2, P/1, Scope2/1
  [Voq] -> Product3/1
  Iabc_s0/1 -> " "/2, abc to dq3/1
  Iabc_s2/1 -> abc to dq4/1
  [Iod] -> Product/2
  [Vod] -> Product1/1
  Selector/1 -> Vodq/1, Demux/1, Scope/1
  [Voq] -> Product2/1
  abc to dq4/1 -> Selector2/1
  [Vod] -> Product/1
  Demux/1 -> [Vod]
  Vabc_s0/1 -> " "/1, abc to dq0/1
  Mux2/1 -> True Q/1
  Fcn/1 -> Vrms/1
  Add1/1 -> Mux2/2, Q/1, Scope3/1
  Mux1/1 -> True P/1
  Selector1/1 -> Demux1/1, Scope1/1
  abc to dq3/1 -> Selector1/1
  Product3/1 -> Gain5/1
  [Ioq] -> Product1/2
  [Iod] -> Product3/2
  Product1/1 -> Gain4/1
  Demux1/2 -> [Ioq]
  Demux1/1 -> [Iod]
  Demux/2 -> [Voq]
  Mux/1 -> True/1
  [Ioq] -> Product2/2
  Selector2/1 -> Icdq/1
  Product2/1 -> Gain3/1
  Product/1 -> Gain1/1
  " "/2 -> Gain2/1
  " "/1 -> Gain/1
  Gain/1 -> Mux1/1, Mux/1
  Gain2/1 -> Mux2/1, Mux/2
  Gain1/1 -> Add2/1
  Gain3/1 -> Add2/2
  Gain4/1 -> Add1/1
  Gain5/1 -> Add1/2

== system simulation_model_constcurrent/Area 3/INVERTER 8/GFM8/Subsystem3 ==
  theta : Inport
  Vabc : Inport  Port=2
  Iabc : Inport  Port=3
  abc to dq1 : spsabctodq0Lib/abc to dq0  Alignment=Aligned with phase A axis
  abc to dq2 : spsabctodq0Lib/abc to dq0  Alignment=Aligned with phase A axis
  Vdq0 : Outport
  Idq0 : Outport  Port=2
  wires:
  Iabc/1 -> abc to dq2/1
  theta/1 -> abc to dq2/2, abc to dq1/2
  abc to dq1/1 -> Vdq0/1
  Vabc/1 -> abc to dq1/1
  abc to dq2/1 -> Idq0/1

== system simulation_model_constcurrent/Area 3/INVERTER 8/GFM8/VSM control ==
  P : Inport
  P_set : Inport  Port=2
  Q : Inport  Port=3
  Q_set : Inport  Port=4
  Clock : Clock
  Clock1 : Clock
  Constant : Constant  Value=2*pi*fbnorm
  Constant1 : Constant  Value=0
  Constant2 : Constant  Value=Vbnorm/sqrt(3)*sqrt(2)
  Constant3 : Constant  Value=2*pi
  Constant5 : Constant  Value=2*pi*fbnorm
  Constant6 : Constant  Value=VSM(8)
  First-Order Filter : spsFirstOrderFilterLib/First-Order Filter  FilterType=Lowpass  Tc=0.08  Ts=0  Initialize=on  Vac_Init=[0, 0, 0]  Vdc_Init=wb  PlotResponse=off  FreqRange="[0,  200,  1]"
  First-Order Filter1 : spsFirstOrderFilterLib/First-Order Filter  FilterType=Lowpass  Tc=0.01  Ts=0  Initialize=on  Vac_Init=[0, 0, 0]  Vdc_Init=Vbnorm/sqrt(3)*sqrt(2)  PlotResponse=off  FreqRange="[0,  200,  1]"
  Gain : Gain  Gain=1/Dq
  Gain1 : Gain  Gain=Dp
  Gain2 : Gain  Gain=D_p_gfm_s(8)
  Gain4 : Gain  Gain=1/Dp
  Gain5 : Gain  Gain=1/D_p_gfm_s(8)
  Gain6 : Gain  Gain=1/J
  Integrator : Integrator  InitialCondition=2*pi*fbnorm
  Integrator1 : Integrator
  Integrator2 : Integrator  InitialCondition=InitialV.theta0
  Mod : Math  Operator=mod
  Multiport Switch : MultiPortSwitch  Inputs=2  SaturateOnIntegerOverflow=off  InputSameDT=off
  Mux : Mux  Inputs=2
  Sum : Sum  Inputs=-|+|-
  Sum1 : Sum  Inputs=-|+
  Sum2 : Sum  Inputs=-+
  Sum3 : Sum  Inputs=+-|
  Sum4 : Sum  Inputs=-|+
  Sum5 : Sum  Inputs=+-|
  Switch : Switch  Threshold=t_gfm  SaturateOnIntegerOverflow=off  InputSameDT=off
  Switch1 : Switch  Threshold=t_gfm  SaturateOnIntegerOverflow=off  InputSameDT=off
  w_ref : Outport  VectorParamsAs1DForOutWhenUnconnected=off
  theta_ref : Outport  Port=2  VectorParamsAs1DForOutWhenUnconnected=off
  Vodq_ref : Outport  Port=3  VectorParamsAs1DForOutWhenUnconnected=off
  theta_output : Outport  Port=4
  theta0 : Outport  Port=5
  wires:
  Constant/1 -> Sum2/1
  Sum/1 -> Gain6/1
  Switch/1 -> [d_output]
  [d_output] -> Sum/1
  Constant2/1 -> Sum3/1
  Mod/1 -> theta_ref/1
  Multiport Switch/1 -> [switch_w]
  Q_set/1 -> Sum1/1
  Mux/1 -> Vodq_ref/1
  Q/1 -> Sum1/2
  Sum1/1 -> Gain/1
  Gain2/1 -> Switch/1
  Integrator2/1 -> theta_output/1, Mod/1  "theta"
  Integrator/1 -> Sum2/2, [vsm_output]  "w"
  Sum2/1 -> [d_input], Integrator1/1
  Constant3/1 -> Mod/2
  Clock/1 -> Switch/2
  [d_output1] -> Sum5/2
  [d_input] -> Gain2/1
  [d_input] -> Gain1/1
  [droop_output] -> Multiport Switch/3
  Sum3/1 -> First-Order Filter1/1
  Constant5/1 -> Sum5/1
  Sum4/1 -> [d_input1]
  Gain6/1 -> Integrator/1
  P_set/1 -> Sum4/1, Sum/2
  Integrator1/1 -> theta0/1
  Constant1/1 -> Mux/2
  Sum5/1 -> First-Order Filter/1
  [vsm_output] -> Multiport Switch/2
  Gain1/1 -> Switch/3
  [switch_w] -> Integrator2/1, w_ref/1
  P/1 -> Sum4/2, Sum/3
  Constant6/1 -> Multiport Switch/1
  First-Order Filter/1 -> [droop_output]
  Gain4/1 -> Switch1/3
  Clock1/1 -> Switch1/2
  [d_input1] -> Gain4/1
  Gain5/1 -> Switch1/1
  Switch1/1 -> [d_output1]
  [d_input1] -> Gain5/1
  Gain/1 -> Sum3/2
  First-Order Filter1/1 -> Mux/1

== system simulation_model_constcurrent/Area 3/INVERTER 8/GFM8/Voltage Loop ==
  v_ref_dq : Inport
  vo_dq : Inport  Port=2
  Demux : Demux  Outputs=2
  Demux1 : Demux  Outputs=2
  Mux : Mux  Inputs=2
  PID Controller : slpidlib/PID Controller  Controller=PI  Form=Parallel  TimeDomain=Continuous-time  UseExternalTs=off  SampleTime=-1  IntegratorMethod=Forward Euler  FilterMethod=Forward Euler  ControllerParametersSource=internal  P=Voltage_P  I=Voltage_I  UseKiTs=off  D=0  UseExternalDerivativeSource=off  N=100  UseFilter=on  TunerSelectOption=Transfer Function Based (PID Tuner App)  InitialConditionSource=internal  InitialConditionForIntegrator=InitialV.Icd  InitialConditionForFilter=0  DifferentiatorICPrevScaledInput=0  ExternalReset=none  TrackingMode=off  Kt=1  LimitOutput=off  SatLimitsSource=internal  UpperSaturationLimit=inf  LowerSaturationLimit=-inf  LinearizeAsGain=on  AntiWindupMode=none  Kb=1  LimitIntegrator=off  UpperIntegratorSaturationLimit=inf  LowerIntegratorSaturationLimit=-inf  POutMin=[]  POutMax=[]  IOutMin=[]  IOutMax=[]  DOutMin=[]  DOutMax=[]  NOutMin=[]  NOutMax=[]  SumOutMin=[]  SumOutMax=[]  SaturationOutMin=[]  SaturationOutMax=[]  PParamMin=[]  PParamMax=[]  IParamMin=[]  IParamMax=[]  DParamMin=[]  DParamMax=[]  NParamMin=[]  NParamMax=[]  KbParamMin=[]  KbParamMax=[]  KtParamMin=[]  KtParamMax=[]  KbOutMin=[]  KbOutMax=[]  KtOutMin=[]  KtOutMax=[]  IntegratorOutMin=[]  IntegratorOutMax=[]  FilterOutMin=[]  FilterOutMax=[]  SumI1OutMin=[]  SumI1OutMax=[]  SumI2OutMin=[]  SumI2OutMax=[]  SumI3OutMin=[]  SumI3OutMax=[]  SumI4OutMin=[]  SumI4OutMax=[]  SumDOutMin=[]  SumDOutMax=[]  DifferentiatorOutMin=[]  DifferentiatorOutMax=[]  FilterDiffOutCoefMin=[]  FilterDiffOutCoefMax=[]  ReciprocalOutMin=[]  ReciprocalOutMax=[]  SumDenOutMin=[]  SumDenOutMax=[]  SumNumOutMin=[]  SumNumOutMax=[]  DivideOutMin=[]  DivideOutMax=[]  UdiffTsProdOutMin=[]  UdiffTsProdOutMax=[]  NTsProdOutMin=[]  NTsProdOutMax=[]  UintegralTsProdOutMin=[]  UintegralTsProdOutMax=[]  UngainTsProdOutMin=[]  UngainTsProdOutMax=[]  ClampingZeroOutDataTypeStr=Inherit: Inherit via back propagation  ClampingZeroOutMin=[]  ClampingZeroOutMax=[]  FilterDenConstantOutDataTypeStr=Inherit: Inherit via back propagation  FilterDenConstantOutMin=[]  FilterDenConstantOutMax=[]  PCopyOutDataTypeStr=Inherit: Inherit via back propagation  PCopyOutMin=[]  PCopyOutMax=[]  NCopyOutDataTypeStr=Inherit: Inherit via back propagation  NCopyOutMin=[]  NCopyOutMax=[]  IntegratorContinuousStateAttributes=''  IntegratorStateMustResolveToSignalObject=off  IntegratorRTWStateStorageClass=Auto  FilterContinuousStateAttributes=''  FilterStateMustResolveToSignalObject=off  FilterRTWStateStorageClass=Auto  ParallelPVariant=InternalParameters  IdealPVariant=Disabled  IVariant=InternalParameters  DVariant=Disabled  IntegratorVariant=Continuous  SatVariant=Disabled  AWVariant=Passthrough  PCopyVariant=Disabled  TRVariant=Disabled  FdbkBlocksVariant=Forward  IdealPFdbkVariant=Disabled  SatFdbkVariant=Disabled  DerivativeFilterVariant=Disabled  NVariant=Disabled  NCopyVariant=Disabled_SignalSpec  FilterICVariant=Disabled  IntegratorICVariant=InternalICs  ExternalResetVariant=Disabled  TRSumVariant=Passthrough  SumFdbkVariant=Disabled  SumVariant=Sum_PI  TsampFilterVariant=InternalTs  TsampNgainVariant=Passthrough  TsampIntegralVariant=Disabled_SignalSpec  ExternalSaturationOutDataTypeStr=Inherit: Same as second input  DerivativeSourceVariant=Disabled  PreIntVariant=InternalPreInt
  PID Controller1 : slpidlib/PID Controller  Controller=PI  Form=Parallel  TimeDomain=Continuous-time  UseExternalTs=off  SampleTime=-1  IntegratorMethod=Forward Euler  FilterMethod=Forward Euler  ControllerParametersSource=internal  P=Voltage_P  I=Voltage_I  UseKiTs=off  D=0  UseExternalDerivativeSource=off  N=100  UseFilter=on  TunerSelectOption=Transfer Function Based (PID Tuner App)  InitialConditionSource=internal  InitialConditionForIntegrator=InitialV.Icq  InitialConditionForFilter=0  DifferentiatorICPrevScaledInput=0  ExternalReset=none  TrackingMode=off  Kt=1  LimitOutput=off  SatLimitsSource=internal  UpperSaturationLimit=inf  LowerSaturationLimit=-inf  LinearizeAsGain=on  AntiWindupMode=none  Kb=1  LimitIntegrator=off  UpperIntegratorSaturationLimit=inf  LowerIntegratorSaturationLimit=-inf  POutMin=[]  POutMax=[]  IOutMin=[]  IOutMax=[]  DOutMin=[]  DOutMax=[]  NOutMin=[]  NOutMax=[]  SumOutMin=[]  SumOutMax=[]  SaturationOutMin=[]  SaturationOutMax=[]  PParamMin=[]  PParamMax=[]  IParamMin=[]  IParamMax=[]  DParamMin=[]  DParamMax=[]  NParamMin=[]  NParamMax=[]  KbParamMin=[]  KbParamMax=[]  KtParamMin=[]  KtParamMax=[]  KbOutMin=[]  KbOutMax=[]  KtOutMin=[]  KtOutMax=[]  IntegratorOutMin=[]  IntegratorOutMax=[]  FilterOutMin=[]  FilterOutMax=[]  SumI1OutMin=[]  SumI1OutMax=[]  SumI2OutMin=[]  SumI2OutMax=[]  SumI3OutMin=[]  SumI3OutMax=[]  SumI4OutMin=[]  SumI4OutMax=[]  SumDOutMin=[]  SumDOutMax=[]  DifferentiatorOutMin=[]  DifferentiatorOutMax=[]  FilterDiffOutCoefMin=[]  FilterDiffOutCoefMax=[]  ReciprocalOutMin=[]  ReciprocalOutMax=[]  SumDenOutMin=[]  SumDenOutMax=[]  SumNumOutMin=[]  SumNumOutMax=[]  DivideOutMin=[]  DivideOutMax=[]  UdiffTsProdOutMin=[]  UdiffTsProdOutMax=[]  NTsProdOutMin=[]  NTsProdOutMax=[]  UintegralTsProdOutMin=[]  UintegralTsProdOutMax=[]  UngainTsProdOutMin=[]  UngainTsProdOutMax=[]  ClampingZeroOutDataTypeStr=Inherit: Inherit via back propagation  ClampingZeroOutMin=[]  ClampingZeroOutMax=[]  FilterDenConstantOutDataTypeStr=Inherit: Inherit via back propagation  FilterDenConstantOutMin=[]  FilterDenConstantOutMax=[]  PCopyOutDataTypeStr=Inherit: Inherit via back propagation  PCopyOutMin=[]  PCopyOutMax=[]  NCopyOutDataTypeStr=Inherit: Inherit via back propagation  NCopyOutMin=[]  NCopyOutMax=[]  IntegratorContinuousStateAttributes=''  IntegratorStateMustResolveToSignalObject=off  IntegratorRTWStateStorageClass=Auto  FilterContinuousStateAttributes=''  FilterStateMustResolveToSignalObject=off  FilterRTWStateStorageClass=Auto  ParallelPVariant=InternalParameters  IdealPVariant=Disabled  IVariant=InternalParameters  DVariant=Disabled  IntegratorVariant=Continuous  SatVariant=Disabled  AWVariant=Passthrough  PCopyVariant=Disabled  TRVariant=Disabled  FdbkBlocksVariant=Forward  IdealPFdbkVariant=Disabled  SatFdbkVariant=Disabled  DerivativeFilterVariant=Disabled  NVariant=Disabled  NCopyVariant=Disabled_SignalSpec  FilterICVariant=Disabled  IntegratorICVariant=InternalICs  ExternalResetVariant=Disabled  TRSumVariant=Passthrough  SumFdbkVariant=Disabled  SumVariant=Sum_PI  TsampFilterVariant=InternalTs  TsampNgainVariant=Passthrough  TsampIntegralVariant=Disabled_SignalSpec  ExternalSaturationOutDataTypeStr=Inherit: Same as second input  DerivativeSourceVariant=Disabled  PreIntVariant=InternalPreInt
  Sum : Sum  Inputs=|+-
  Sum1 : Sum  Inputs=|+-
  i_ref_dq : Outport  VectorParamsAs1DForOutWhenUnconnected=off
  wires:
  Mux/1 -> i_ref_dq/1
  v_ref_dq/1 -> Demux/1
  vo_dq/1 -> Demux1/1
  Demux/1 -> [vo_ref_d]
  Demux/2 -> [vo_ref_q]
  Demux1/1 -> [vo_d]
  Demux1/2 -> [vo_q]
  Sum/1 -> PID Controller/1
  [vo_d] -> Sum/2
  Sum1/1 -> PID Controller1/1
  [vo_q] -> Sum1/2
  PID Controller/1 -> Mux/1
  PID Controller1/1 -> Mux/2
  [vo_ref_d] -> Sum/1
  [vo_ref_q] -> Sum1/1
